simulink model "Portable_Charging_System_Test_2"  (R2025b)
settings: Solver=ode23t  StartTime=0.0  StopTime=11  RelTol=1e-3
libraries: fl_lib x49, nesl_utility x12, ee_lib x3, slpidlib x2, batteryecm_lib x2, eePwmGenerator x1
(part 2 of 2)

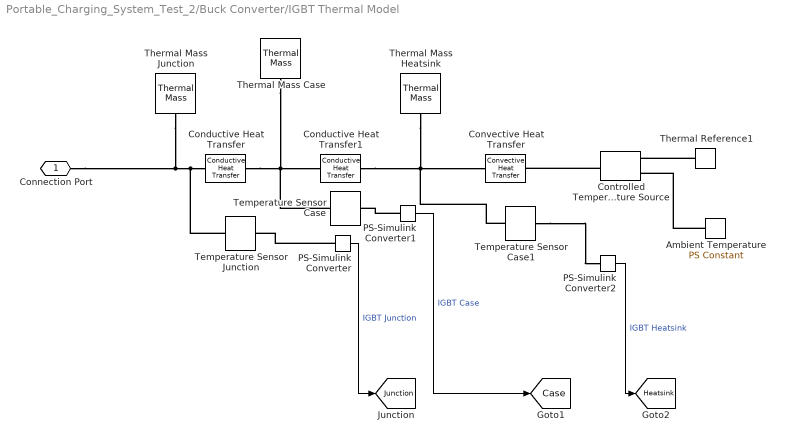
== system Portable_Charging_System_Test_2/Buck Converter/IGBT Thermal Model ==
  Ambient Temperature : fl_lib/Physical Signals/Sources/PS Constant  constant=298.15
  Conductive Heat Transfer : fl_lib/Thermal/Thermal Elements/Conductive Heat Transfer  thermal_type=foundation.enum.ConstantVariableTabulated.Constant  wall_geometry=foundation.enum.ConductionWallGeometry.Planar  area=5 m^2  thickness=360 m  d_in=0.05 m  d_out=0.1 m  L=1 m  th_cond_min=10 W/(K*m)  th_cond=150 W/(K*m)  th_cond_TLU=[413, 401, 392, 383, 371, 357, 342] W/(K*m)  temp_TLU=[200, 273, 400, 600, 800, 1000, 1200] K  T_specify=off  T_priority=None  T=0 K  T_nominal_specify=off  T_nominal_value=1  T_nominal_unit=K  Q_specify=off  Q_priority=None  Q=0 W  Q_nominal_specify=off  Q_nominal_value=1  Q_nominal_unit=W
  Conductive Heat Transfer1 : fl_lib/Thermal/Thermal Elements/Conductive Heat Transfer  thermal_type=foundation.enum.ConstantVariableTabulated.Constant  wall_geometry=foundation.enum.ConductionWallGeometry.Planar  area=14 m^2  thickness=0.1 m  d_in=0.05 m  d_out=0.1 m  L=1 m  th_cond_min=10 W/(K*m)  th_cond=3 W/(K*m)  th_cond_TLU=[413, 401, 392, 383, 371, 357, 342] W/(K*m)  temp_TLU=[200, 273, 400, 600, 800, 1000, 1200] K  T_specify=off  T_priority=None  T=0 K  T_nominal_specify=off  T_nominal_value=1  T_nominal_unit=K  Q_specify=off  Q_priority=None  Q=0 W  Q_nominal_specify=off  Q_nominal_value=1  Q_nominal_unit=W
  Controlled Temperature Source : fl_lib/Thermal/Thermal Sources/Controlled Temperature Source
  Convective Heat Transfer : fl_lib/Thermal/Thermal Elements/Convective Heat Transfer  thermal_type=foundation.enum.constant_variable.constant  area=40 m^2  heat_tr_coeff=20 W/(K*m^2)  min_heat_tr_coeff=1e-3 W/(K*m^2)  T_specify=off  T_priority=None  T=0 K  T_nominal_specify=off  T_nominal_value=1  T_nominal_unit=K  Q_specify=off  Q_priority=None  Q=0 W  Q_nominal_specify=off  Q_nominal_value=1  Q_nominal_unit=W
  PS-Simulink Converter : nesl_utility/PS-Simulink Converter  PhysicalDomain=network_engine_domain  SubClassName=ps_output  LeftPortType=input  RightPortType=output  PseudoPeriodic=off  Frequencies=[]  VectorFormat=inherit  Unit=inherit  AffineConversion=off
  PS-Simulink Converter1 : nesl_utility/PS-Simulink Converter  PhysicalDomain=network_engine_domain  SubClassName=ps_output  LeftPortType=input  RightPortType=output  PseudoPeriodic=off  Frequencies=[]  VectorFormat=inherit  Unit=inherit  AffineConversion=off
  PS-Simulink Converter2 : nesl_utility/PS-Simulink Converter  PhysicalDomain=network_engine_domain  SubClassName=ps_output  LeftPortType=input  RightPortType=output  PseudoPeriodic=off  Frequencies=[]  VectorFormat=inherit  Unit=inherit  AffineConversion=off
  Temperature Sensor Case : fl_lib/Thermal/Thermal Sensors/Temperature Sensor  temperature_measure=foundation.enum.MeasurementReference.absolute
      settings: InternalSimscapePortConfiguration="{\"Bottom\":[],\"Left\":[{\"id\":\"A\",\"label\":\"A\",\"type\":\"foundation.thermal.thermal\"}],\"Right\":[{\"id\":\"T\",\"label\":\"T\",\"type\":\"output\"}],\"Top\":[]}"
  Temperature Sensor Case1 : fl_lib/Thermal/Thermal Sensors/Temperature Sensor  temperature_measure=foundation.enum.MeasurementReference.absolute
      settings: InternalSimscapePortConfiguration="{\"Bottom\":[],\"Left\":[{\"id\":\"A\",\"label\":\"A\",\"type\":\"foundation.thermal.thermal\"}],\"Right\":[{\"id\":\"T\",\"label\":\"T\",\"type\":\"output\"}],\"Top\":[]}"
  Temperature Sensor Junction : fl_lib/Thermal/Thermal Sensors/Temperature Sensor  temperature_measure=foundation.enum.MeasurementReference.absolute
      settings: InternalSimscapePortConfiguration="{\"Bottom\":[],\"Left\":[{\"id\":\"A\",\"label\":\"A\",\"type\":\"foundation.thermal.thermal\"}],\"Right\":[{\"id\":\"T\",\"label\":\"T\",\"type\":\"output\"}],\"Top\":[]}"
  Thermal Mass Case : fl_lib/Thermal/Thermal Elements/Thermal Mass  mass_type=foundation.enum.constant_variable.constant  mass=0.02 kg  sp_heat=385 J/(K*kg)  mass_min=1e-6 kg  num_ports=foundation.enum.numPorts2.one  m_specify=off  m_priority=High  m=1 kg  m_nominal_specify=off  m_nominal_value=1  m_nominal_unit=kg  T_specify=on  T_priority=High  T=298.15 K  T_nominal_specify=off  T_nominal_value=1  T_nominal_unit=K  Q_specify=off  Q_priority=None  Q=0 W  Q_nominal_specify=off  Q_nominal_value=1  Q_nominal_unit=W
  Thermal Mass Heatsink : fl_lib/Thermal/Thermal Elements/Thermal Mass  mass_type=foundation.enum.constant_variable.constant  mass=0.2 kg  sp_heat=900 J/(K*kg)  mass_min=1e-6 kg  num_ports=foundation.enum.numPorts2.one  m_specify=off  m_priority=High  m=1 kg  m_nominal_specify=off  m_nominal_value=1  m_nominal_unit=kg  T_specify=on  T_priority=High  T=298.15 K  T_nominal_specify=off  T_nominal_value=1  T_nominal_unit=K  Q_specify=off  Q_priority=None  Q=0 W  Q_nominal_specify=off  Q_nominal_value=1  Q_nominal_unit=W
  Thermal Mass Junction : fl_lib/Thermal/Thermal Elements/Thermal Mass  mass_type=foundation.enum.constant_variable.constant  mass=0.001 kg  sp_heat=700 J/(K*kg)  mass_min=1e-6 kg  num_ports=foundation.enum.numPorts2.one  m_specify=off  m_priority=High  m=1 kg  m_nominal_specify=off  m_nominal_value=1  m_nominal_unit=kg  T_specify=on  T_priority=High  T="298.15  K"  T_nominal_specify=off  T_nominal_value=1  T_nominal_unit=K  Q_specify=off  Q_priority=None  Q=0 W  Q_nominal_specify=off  Q_nominal_value=1  Q_nominal_unit=W
  Thermal Reference1 : fl_lib/Thermal/Thermal Elements/Thermal Reference
  Connection Port : PMIOPort  Side=Left
  tag scope: Case=global, Heatsink=global, Junction=global
  wires:
  PS-Simulink Converter/1 -> [Junction]  "IGBT Junction"
  PS-Simulink Converter1/1 -> [Case]  "IGBT Case"
  PS-Simulink Converter2/1 -> [Heatsink]  "IGBT Heatsink"
  connections:
  Conductive Heat Transfer1/RConn1 -- Temperature Sensor Case1/LConn1 -- Thermal Mass Heatsink/LConn1 -- Convective Heat Transfer/LConn1
  Conductive Heat Transfer/RConn1 -- Thermal Mass Case/LConn1 -- Temperature Sensor Case/LConn1 -- Conductive Heat Transfer1/LConn1
  Connection Port/RConn1 -- Thermal Mass Junction/LConn1 -- Temperature Sensor Junction/LConn1 -- Conductive Heat Transfer/LConn1
  Controlled Temperature Source/LConn1 -- Convective Heat Transfer/RConn1
  Thermal Reference1/LConn1 -- Controlled Temperature Source/RConn2
  PS-Simulink Converter/LConn1 -- Temperature Sensor Junction/RConn1
  Ambient Temperature/RConn1 -- Controlled Temperature Source/RConn1
  PS-Simulink Converter1/LConn1 -- Temperature Sensor Case/RConn1
  Temperature Sensor Case1/RConn1 -- PS-Simulink Converter2/LConn1

== system Portable_Charging_System_Test_2/Input Measurements & Analysis/SOC Coulomb Counting ==
  socOutCell : Inport
  Constant2 : Constant  Value=6.28
  Constant3 : Constant  Value=3600
  Divide : Product  Inputs=*/
  Gain : Gain  Gain=100
  Product : Product
  Out1 : Outport
  wires:
  Constant3/1 -> Product/1
  Product/1 -> Divide/2
  socOutCell/1 -> Divide/1
  Gain/1 -> Out1/1
  Constant2/1 -> Product/2
  Divide/1 -> Gain/1

== system Portable_Charging_System_Test_2/Output Measurements & Analysis/SOC Coulomb Counting ==
  socOutCell : Inport
  Constant2 : Constant  Value=309
  Constant3 : Constant  Value=3600
  Divide : Product  Inputs=*/
  Gain : Gain  Gain=100
  Product : Product
  Out1 : Outport
  wires:
  Product/1 -> Divide/2
  Constant2/1 -> Product/2
  Constant3/1 -> Product/1
  Gain/1 -> Out1/1
  socOutCell/1 -> Divide/1
  Divide/1 -> Gain/1

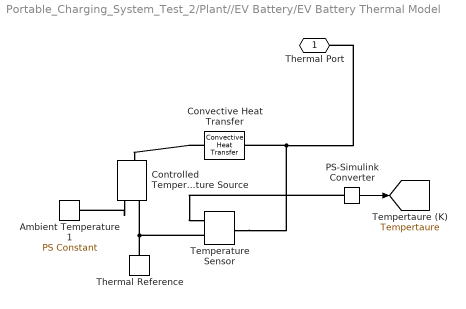
== system Portable_Charging_System_Test_2/Plant//EV Battery/EV Battery Thermal Model ==
  Ambient Temperature1 : fl_lib/Physical Signals/Sources/PS Constant  constant=292.15
  Controlled Temperature Source : fl_lib/Thermal/Thermal Sources/Controlled Temperature Source
  Convective Heat Transfer : fl_lib/Thermal/Thermal Elements/Convective Heat Transfer  thermal_type=foundation.enum.constant_variable.constant  area=1e-4 m^2  heat_tr_coeff=20 W/(K*m^2)  min_heat_tr_coeff=1e-3 W/(K*m^2)  T_specify=off  T_priority=None  T=0 K  T_nominal_specify=off  T_nominal_value=1  T_nominal_unit=K  Q_specify=off  Q_priority=None  Q=0 W  Q_nominal_specify=off  Q_nominal_value=1  Q_nominal_unit=W
  PS-Simulink Converter : nesl_utility/PS-Simulink Converter  PhysicalDomain=network_engine_domain  SubClassName=ps_output  LeftPortType=input  RightPortType=output  PseudoPeriodic=off  Frequencies=[]  VectorFormat=inherit  Unit=inherit  AffineConversion=off
  Temperature Sensor : fl_lib/Thermal/Thermal Sensors/Temperature Sensor  temperature_measure=foundation.enum.MeasurementReference.difference
  Thermal Reference : fl_lib/Thermal/Thermal Elements/Thermal Reference
  Thermal Port : PMIOPort  Side=Left
  tag scope: Tempertaure=global
  wires:
  PS-Simulink Converter/1 -> [Tempertaure]
  connections:
  Temperature Sensor/LConn1 -- Thermal Port/RConn1 -- Convective Heat Transfer/LConn1
  Convective Heat Transfer/RConn1 -- Controlled Temperature Source/LConn1
  Temperature Sensor/RConn1 -- Controlled Temperature Source/RConn2 -- Thermal Reference/LConn1
  Controlled Temperature Source/RConn1 -- Ambient Temperature1/RConn1
  PS-Simulink Converter/LConn1 -- Temperature Sensor/RConn2

== stateflow chart Portable_Charging_System_Test_2/Current Termination Logic ==
  state Charging
    during:
    Iref_out = Iref_in;
    Charge_Enable = 1;
  state Charge_Finish
    during:
    Charge_Enable = 0;
  (default) -> Charging
  Charging -> Charge_Finish : [Mode == 1 && Icharge <= 30.9]
  data: Iref_out output double size=1; Charge_Enable output; Icharge input; Iref_in input double size=1; Mode input

== stateflow chart Portable_Charging_System_Test_2/CC-CV Logic ==
  state CC
    during:
    Mode = 0;
  state CV
    during:
    Mode = 1;
  (default) -> CC
  CC -> CV : [Vout >= 294.35]
  data: Vout input; Mode output double
